simulink model "receive_a429"  (R2020b)
settings: Solver=FixedStepDiscrete  StartTime=0.0  StopTime=10.0  RelTol=1e-3
model workspace (MAT data in the model file):
  ED247Configuration.ECICFile = 'Z:\ED247\ed247_for_simulink\doc\examples\receiveA429\ecic_func_exchange_a429_uc_tester_simple.xml'
  ED247Configuration.ICDFiles = {'Z:\ED247\ed247_for_simulink\doc\examples\receiveA429\icd_func_exchange_a429_uc_tester_simple.xml'}
  ED247Configuration.Configuration(1).name = 'T11M4_A429_SIMU2SWIM_BUS_1_350_10'
  ED247Configuration.Configuration(1).direction = 'IN'
  ED247Configuration.Configuration(1).type = 'uint8'
  ED247Configuration.Configuration(1).dimensions = 1
  ED247Configuration.Configuration(1).width = 4
  ED247Configuration.Configuration(1).size = 4
  ED247Configuration.Configuration(1).sample_time = 1
  ED247Configuration.Configuration(1).validity_duration = 1
  ED247Configuration.Configuration(1).signal_type = 'A429'
  ED247Configuration.Configuration(1).sample_size = 4
  ED247Configuration.Configuration(2).name = 'T11M4_A429_SIMU2SWIM_BUS_1_200_10'
  ED247Configuration.Configuration(2).direction = 'IN'
  ED247Configuration.Configuration(2).type = 'uint8'
  ED247Configuration.Configuration(2).dimensions = 1
  ED247Configuration.Configuration(2).width = 4
  ED247Configuration.Configuration(2).size = 4
  ED247Configuration.Configuration(2).sample_time = 1
  ED247Configuration.Configuration(2).validity_duration = 2
  ED247Configuration.Configuration(2).signal_type = 'A429'
  ED247Configuration.Configuration(2).sample_size = 4
  ED247Configuration.Configuration(3).name = 'T11M4_A429_SIMU2SWIM_BUS_1_200_11'
  ED247Configuration.Configuration(3).direction = 'IN'
  ED247Configuration.Configuration(3).type = 'uint8'
  ED247Configuration.Configuration(3).dimensions = 1
  ED247Configuration.Configuration(3).width = 4
  ED247Configuration.Configuration(3).size = 4
  ED247Configuration.Configuration(3).sample_time = 1
  ED247Configuration.Configuration(3).validity_duration = 3
  ED247Configuration.Configuration(3).signal_type = 'A429'
  ED247Configuration.Configuration(3).sample_size = 4
libraries: lib_ed247 x2
settings Model: Creator=odufour  LastModifiedBy=odufour
settings OptimizationCC: DefaultParameterBehavior=Inlined  EnhancedBackFolding=on  PassReuseOutputArgsAs=Individual arguments  ZeroExternalMemoryAtStartup=off  ZeroInternalMemoryAtStartup=off  EfficientTunableParamExpr=on
settings DebuggingCC: InheritedTsInSrcMsg=none  ParameterTunabilityLossMsg=error  ArithmeticOperatorsInVariantConditions=warning
settings SFSimCC: MATLABDynamicMemAlloc=off  CustomCodeUndefinedFunction=UseInterfaceOnly
settings RTWCC: Description=Embedded Coder  SystemTargetFile=ert.tlc  GenCodeOnly=on  TemplateMakefile=ert_default_tmf  GenerateReport=on  IncludeHyperlinkInReport=on  GenerateTraceInfo=on  GenerateTraceReport=on  GenerateTraceReportSl=on  GenerateTraceReportSf=on  GenerateTraceReportEml=on
settings CodeAppCC: ForceParamTrailComments=on  IgnoreCustomStorageClasses=off  OperatorAnnotations=on  SimulinkDataObjDesc=on  SFDataObjDesc=on  InsertBlockDesc=on  StateflowObjectComments=on
settings ERTTargetCC: TargetLangStandard=C99 (ISO)  GenerateSampleERTMain=on  InlinedParameterPlacement=NonHierarchical  ERTCustomFileTemplate=example_file_process.tlc

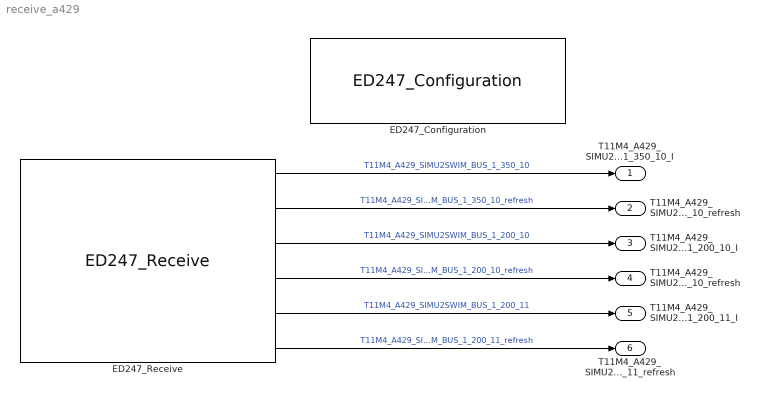
== system receive_a429 ==
  ED247_Configuration : lib_ed247/ED247_Configuration  configurationFilename='ecic_func_exchange_a429_uc_tester_simple.xml'  enableLog=on  logFilename='<PROJECT_FOLDER>\tests\_files\tmp.log'
      settings: SourceProductName=Airbus ED247
  ED247_Receive : lib_ed247/ED247_Receive  enable_refresh=on  refresh_factor=1  sample_time=-1  show_port_labels=on
      settings: SourceProductName=Airbus ED247
  T11M4_A429_SIMU2SWIM_BUS_1_350_10_I : Outport  OutDataTypeStr=uint8  PortDimensions=4  SampleTime=0.1
  T11M4_A429_SIMU2SWIM_BUS_1_350_10_refresh : Outport  Port=2  OutDataTypeStr=boolean  PortDimensions=1  SampleTime=0.1
  T11M4_A429_SIMU2SWIM_BUS_1_200_10_I : Outport  Port=3  OutDataTypeStr=uint8  PortDimensions=4  SampleTime=0.1
  T11M4_A429_SIMU2SWIM_BUS_1_200_10_refresh : Outport  Port=4  OutDataTypeStr=boolean  PortDimensions=1  SampleTime=0.1
  T11M4_A429_SIMU2SWIM_BUS_1_200_11_I : Outport  Port=5  OutDataTypeStr=uint8  PortDimensions=4  SampleTime=0.1
  T11M4_A429_SIMU2SWIM_BUS_1_200_11_refresh : Outport  Port=6  OutDataTypeStr=boolean  PortDimensions=1  SampleTime=0.1
  wires:
  ED247_Receive/2 -> T11M4_A429_SIMU2SWIM_BUS_1_350_10_refresh/1  "T11M4_A429_SIMU2SWIM_BUS_1_350_10_refresh"
  ED247_Receive/1 -> T11M4_A429_SIMU2SWIM_BUS_1_350_10_I/1  "T11M4_A429_SIMU2SWIM_BUS_1_350_10"
  ED247_Receive/4 -> T11M4_A429_SIMU2SWIM_BUS_1_200_10_refresh/1  "T11M4_A429_SIMU2SWIM_BUS_1_200_10_refresh"
  ED247_Receive/3 -> T11M4_A429_SIMU2SWIM_BUS_1_200_10_I/1  "T11M4_A429_SIMU2SWIM_BUS_1_200_10"
  ED247_Receive/6 -> T11M4_A429_SIMU2SWIM_BUS_1_200_11_refresh/1  "T11M4_A429_SIMU2SWIM_BUS_1_200_11_refresh"
  ED247_Receive/5 -> T11M4_A429_SIMU2SWIM_BUS_1_200_11_I/1  "T11M4_A429_SIMU2SWIM_BUS_1_200_11"
